simulink library "apCopterDragonfly_lib"  (R2018b)
settings: Solver=VariableStepAuto  StartTime=0.0  StopTime=10.0  RelTol=1e-3
undefined symbols (not defined in the file or in its folder): ap_dragonfly, DiscIntNeverNeededParam
libraries: simulink x2, cntrlAttiRedIndi_lib x2, cntrlPosNdi_lib x2, indi_lib x1, traj_lib x1, control_allocation_lib x1, ndi_lib x1, filters_lib x1, fmCopterAltHoldIndi_lib x1, axes_transformation_lib x1
settings Model: Creator=Ybeyer  LastModifiedBy=yannic
settings SFSimCC: SimUseLocalCustomCode=off
settings RTWCC: RTWUseLocalCustomCode=off
settings CodeAppCC: StateflowObjectComments=on

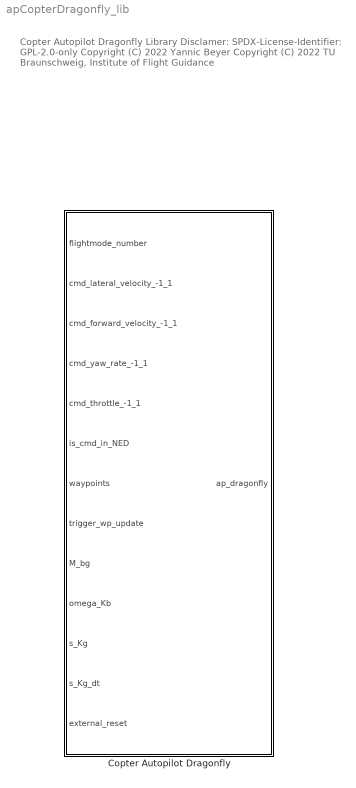
== system apCopterDragonfly_lib ==
  note: Copter Autopilot Dragonfly Library
      |
      | Disclamer:
      | SPDX-License-Identifier: GPL-2.0-only
      |
      | Copyright (C) 2022 Yannic Beyer
      | Copyright (C) 2022 TU Braunschweig, Institute of Flight Guidance
  Copter Autopilot Dragonfly : Subsystem  mask{fm=ap_dragonfly}
      mask prompts: fm "Dragonfly parameters struct, see apCopterDragonflyLoadParams"
      mask DialogControl DescGroupVar Prompt: Copter Autopilot Dragonfly
      mask DialogControl Control1 Prompt: flightmode numbers:
      mask DialogControl Control2 Prompt: loiter: 0
      mask DialogControl Control3 Prompt: guided: 1

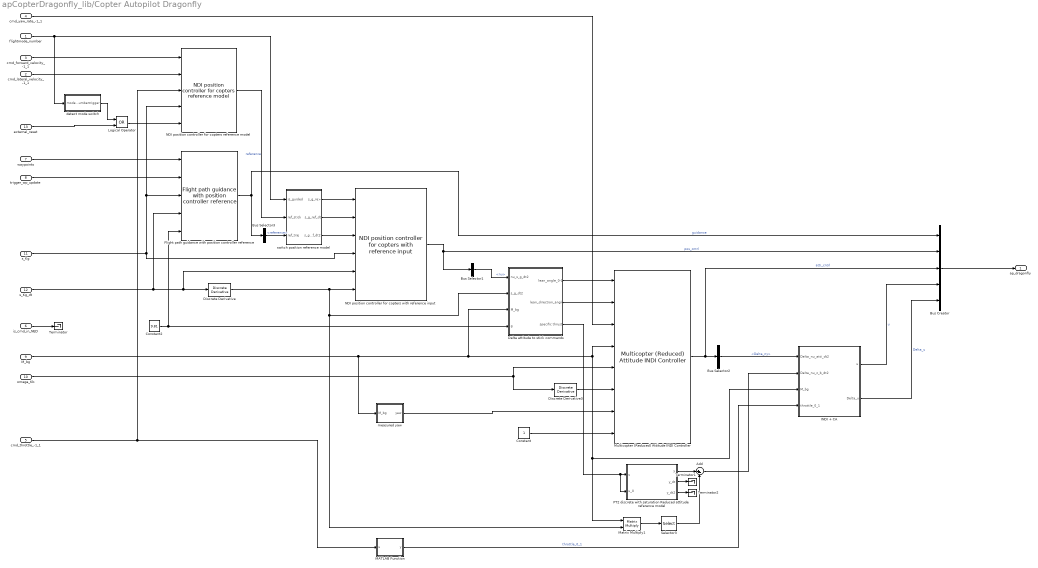
== system apCopterDragonfly_lib/Copter Autopilot Dragonfly ==
  flightmode_number : Inport  SampleTime=fm.sample_time
  cmd_lateral_velocity_-1_1 : Inport  Port=2  SampleTime=fm.sample_time
  cmd_forward_velocity_-1_1 : Inport  Port=3  SampleTime=fm.sample_time
  cmd_yaw_rate_-1_1 : Inport  Port=4  SampleTime=fm.sample_time
  cmd_throttle_-1_1 : Inport  Port=5  SampleTime=fm.sample_time
  is_cmd_in_NED : Inport  Port=6  SampleTime=fm.sample_time
  waypoints : Inport  Port=7
  trigger_wp_update : Inport  Port=8
  M_bg : Inport  Port=9  SampleTime=fm.sample_time
  omega_Kb : Inport  Port=10  SampleTime=fm.sample_time
  s_Kg : Inport  Port=11  SampleTime=fm.sample_time
  s_Kg_dt : Inport  Port=12  SampleTime=fm.sample_time
  external_reset : Inport  Port=13  SampleTime=fm.sample_time
  Add : Sum  Inputs=|+-
  Bus Creator : BusCreator  Inputs=5
  Bus Selector1 : BusSelector  OutputSignals=pseudo_control.nu
  Bus Selector2 : BusSelector  OutputSignals=pseudo_control.Delta_ny
  Bus Selector3 : BusSelector  OutputSignals=reference
  Constant : Constant
  Constant2 : Constant  Value=9.81
  Delta attitude to stick commands : Subsystem
  Discrete Derivative : simulink/Discrete/Discrete Derivative  gainval=1.0  ICPrevScaledInput=0.0  OutMin=[]  OutMax=[]  OutDataType=fixdt(1, 16)  OutScaling=2^-10  DoSatur=off
  Discrete Derivative3 : simulink/Discrete/Discrete Derivative  gainval=1.0  ICPrevScaledInput=0.0  OutMin=[]  OutMax=[]  OutDataType=fixdt(1, 16)  OutScaling=2^-10  DoSatur=off
  Flight path guidance with position controller reference : traj_lib/Flight path guidance with position controller reference  traj_params=fm.traj  T_inner_loop=2./fm.atc.rm.leanfreq + fm.motor_time_constant + 2./fm.sens_filt.omega
      settings: SourceProductName=LADAC
  INDI + CA : Subsystem
  Logical Operator : Logic  Operator=OR  AllPortsSameDT=off  OutDataTypeStr=boolean
  MATLAB Function : MATLAB Function  TreatAsAtomicUnit=on
  Matrix Multiply1 : Product  Multiplication=Matrix(*)
  Multicopter (Reduced) Attitude INDI Controller : cntrlAttiRedIndi_lib/Multicopter (Reduced) Attitude INDI Controller  atc=fm.atc  T=fm.motor_time_constant + 2./fm.sens_filt.omega
  NDI position controller for copters reference model : cntrlPosNdi_lib/NDI position controller for copters reference model  psc=fm.psc
      settings: SourceProductName=LADAC
  NDI position controller for copters with reference input : cntrlPosNdi_lib/NDI position controller for copters with reference input  psc=fm.psc  T_inner_loop=2./fm.atc.rm.leanfreq + fm.motor_time_constant + 2./fm.sens_filt.omega
      settings: SourceProductName=LADAC
  PT2 discrete with saturation Reduced attitude reference model : Subsystem  mask{omega=fm.atc.rm.leanfreq, d=fm.atc.rm.leandamp, x_dt2_max=inf, x_dt2_min=-inf, x_dt_max=inf, x_dt_min=-inf, x_max=inf, x_min=-inf, x_init=0, x_dt_init=0}
      mask prompts: omega "Natural frequency"; d "Damping ratio"; x_dt2_max "Maximum acceleration"; x_dt2_min "Minimum acceleration"; x_dt_max "Maximum rate"; x_dt_min "Minimum rate"; x_max "Maximum position"; x_min "Minimum position"; x_init "Initial position"; x_dt_init "Initial rate"
  Selector3 : Selector  InputPortWidth=3  IndexOptions=Index vector (dialog)  Indices=3  OutputSizes=1
  Terminator : Terminator
  Terminator1 : Terminator
  Terminator2 : Terminator
  detect mode switch : Subsystem
  measured yaw : Subsystem
  switch position reference model : Subsystem
  ap_dragonfly : Outport  SampleTime=fm.sample_time
  wires:
  waypoints/1 -> Flight path guidance with position controller reference/1
  cmd_lateral_velocity_-1_1/1 -> NDI position controller for copters reference model/2
  cmd_forward_velocity_-1_1/1 -> NDI position controller for copters reference model/1
  PT2 discrete with saturation Reduced attitude reference model/1(y) -> Add/1
  PT2 discrete with saturation Reduced attitude reference model/3(y_dt2) -> Terminator2/1
  PT2 discrete with saturation Reduced attitude reference model/2(y_dt) -> Terminator1/1
  Add/1 -> INDI + CA/2(Delta_nu_z_b_dt2)
  Bus Selector2/1 -> INDI + CA/1(Delta_nu_atti_dt2)  "<Delta_ny>"
  cmd_throttle_-1_1/1 -> NDI position controller for copters reference model/3, MATLAB Function/1(u)
  INDI + CA/2(Delta_u) -> Bus Creator/5  "Delta_u"
  INDI + CA/1(u) -> Bus Creator/4  "u"
  MATLAB Function/1(y) -> INDI + CA/4(throttle_0_1)  "throttle_0_1"
  Delta attitude to stick commands/1(lean_angle_0-1) -> Multicopter (Reduced) Attitude INDI Controller/1
  Delta attitude to stick commands/2(lean_direction_angle) -> Multicopter (Reduced) Attitude INDI Controller/2
  Discrete Derivative3/1 -> Multicopter (Reduced) Attitude INDI Controller/6
  Multicopter (Reduced) Attitude INDI Controller/1 -> Bus Creator/3, Bus Selector2/1  "atti_cntrl"
  is_cmd_in_NED/1 -> Terminator/1
  Bus Creator/1 -> ap_dragonfly/1
  Bus Selector1/1 -> Delta attitude to stick commands/1(nu_s_g_dt2)  "<nu>"
  measured yaw/1(yaw) -> Multicopter (Reduced) Attitude INDI Controller/7
  M_bg/1 -> measured yaw/1(M_bg), Delta attitude to stick commands/3(M_bg), INDI + CA/3(M_bg), Matrix Multiply1/1, Multicopter (Reduced) Attitude INDI Controller/4
  NDI position controller for copters with reference input/1 -> Bus Selector1/1, Bus Creator/2  "pos_cntrl"
  omega_Kb/1 -> Multicopter (Reduced) Attitude INDI Controller/5, Discrete Derivative3/1
  s_Kg/1 -> NDI position controller for copters reference model/4, Flight path guidance with position controller reference/3, NDI position controller for copters with reference input/4
  Constant/1 -> Multicopter (Reduced) Attitude INDI Controller/8
  cmd_yaw_rate_-1_1/1 -> Multicopter (Reduced) Attitude INDI Controller/3
  s_Kg_dt/1 -> Flight path guidance with position controller reference/4, Discrete Derivative/1, NDI position controller for copters with reference input/5
  Flight path guidance with position controller reference/1 -> Bus Creator/1, Bus Selector3/1  "guidance"
  switch position reference model/3(s_g_ref_dt2) -> NDI position controller for copters with reference input/3
  switch position reference model/2(s_g_ref_dt) -> NDI position controller for copters with reference input/2
  switch position reference model/1(s_g_re>) -> NDI position controller for copters with reference input/1
  Matrix Multiply1/1 -> Selector3/1
  Selector3/1 -> Add/2
  Delta attitude to stick commands/3(specific thrust) -> PT2 discrete with saturation Reduced attitude reference model/2(u_0), PT2 discrete with saturation Reduced attitude reference model/1(u)
  trigger_wp_update/1 -> Flight path guidance with position controller reference/2
  Discrete Derivative/1 -> Matrix Multiply1/2, Delta attitude to stick commands/2(s_g_dt2), NDI position controller for copters with reference input/6
  Constant2/1 -> Flight path guidance with position controller reference/5, Delta attitude to stick commands/4(g)
  NDI position controller for copters reference model/1 -> switch position reference model/2(ref_stick)  "reference"
  Bus Selector3/1 -> switch position reference model/3(ref_traj)  "<reference>"
  flightmode_number/1 -> detect mode switch/1(mode number), switch position reference model/1(is_guided)
  Logical Operator/1 -> NDI position controller for copters reference model/5
  detect mode switch/1(trigger) -> Logical Operator/1
  external_reset/1 -> Logical Operator/2

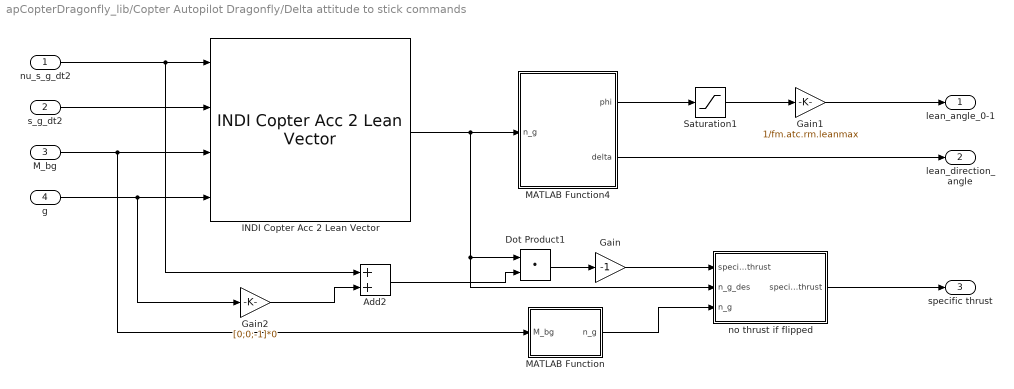
== system apCopterDragonfly_lib/Copter Autopilot Dragonfly/Delta attitude to stick commands ==
  nu_s_g_dt2 : Inport
  s_g_dt2 : Inport  Port=2
  M_bg : Inport  Port=3
  g : Inport  Port=4
  Add2 : Sum
  Dot Product1 : DotProduct  InputSameDT=on  OutDataTypeStr=Inherit: Inherit via internal rule
  Gain : Gain  Gain=-1
  Gain1 : Gain  Gain=1/fm.atc.rm.leanmax
  Gain2 : Gain  Gain=[0;0;-1]*0
  INDI Copter Acc 2 Lean Vector : indi_lib/INDI Copter Acc 2 Lean Vector  SystemSampleTime=-1
      settings: SourceProductName=LADAC
  MATLAB Function : MATLAB Function  TreatAsAtomicUnit=on
  MATLAB Function4 : MATLAB Function  TreatAsAtomicUnit=on
  Saturation1 : Saturate  UpperLimit=fm.atc.rm.leanmax  LowerLimit=0
  no thrust if flipped : MATLAB Function  TreatAsAtomicUnit=on
  lean_angle_0-1 : Outport
  lean_direction_angle : Outport  Port=2
  specific thrust : Outport  Port=3
  wires:
  MATLAB Function4/2(delta) -> lean_direction_angle/1
  Gain1/1 -> lean_angle_0-1/1
  nu_s_g_dt2/1 -> Add2/1, INDI Copter Acc 2 Lean Vector/1
  Saturation1/1 -> Gain1/1
  MATLAB Function4/1(phi) -> Saturation1/1
  g/1 -> Gain2/1, INDI Copter Acc 2 Lean Vector/4
  s_g_dt2/1 -> INDI Copter Acc 2 Lean Vector/2
  M_bg/1 -> MATLAB Function/1(M_bg), INDI Copter Acc 2 Lean Vector/3
  Dot Product1/1 -> Gain/1
  Gain/1 -> no thrust if flipped/1("specific_thrust ")
  INDI Copter Acc 2 Lean Vector/1 -> no thrust if flipped/2(n_g_des), Dot Product1/1, MATLAB Function4/1(n_g)
  Gain2/1 -> Add2/2
  Add2/1 -> Dot Product1/2
  no thrust if flipped/1(specific_thrust) -> specific thrust/1
  MATLAB Function/1(n_g) -> no thrust if flipped/3(n_g)

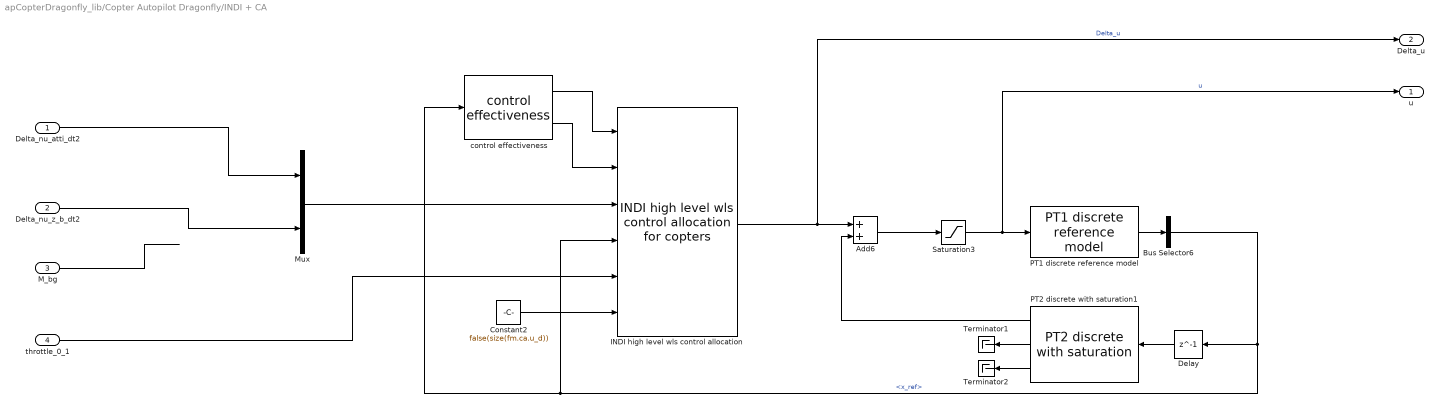
== system apCopterDragonfly_lib/Copter Autopilot Dragonfly/INDI + CA ==
  Delta_nu_atti_dt2 : Inport
  Delta_nu_z_b_dt2 : Inport  Port=2
  M_bg : Inport  Port=3
  throttle_0_1 : Inport  Port=4
  Add6 : Sum
  Bus Selector6 : BusSelector  OutputSignals=x_ref
  Constant2 : Constant  Value=false(size(fm.ca.u_d))
  Delay : Delay  DelayLength=1
  INDI high level wls control allocation : control_allocation_lib/INDI high level wls control allocation for copters  ca=fm.ca  is_Delta_W_v_check=off  is_W_check=off  is_iter_check=off
  Mux : Mux  Inputs=2
  PT1 discrete reference model : ndi_lib/PT1 discrete reference model  T=fm.motor_time_constant  x_max=inf  x_min=-inf  x_dt_max=inf  x_dt_min=-inf  x_init=0
      settings: SourceProductName=LADAC
  PT2 discrete with saturation1 : filters_lib/PT2 discrete with saturation  omega=fm.sens_filt.omega  d=fm.sens_filt.D  x_dt2_max=inf  x_dt2_min=-inf  x_dt_max=inf  x_dt_min=-inf  x_max=inf  x_min=-inf  x_init=0  x_dt_init=0
      settings: SourceProductName=LADAC
  Saturation3 : Saturate  UpperLimit=fm.ca.u_max  LowerLimit=fm.ca.u_min
  Terminator1 : Terminator
  Terminator2 : Terminator
  control effectiveness : fmCopterAltHoldIndi_lib/Multicopter Altitude Hold Flight Mode with INDI and reduced attitude control/control effectiveness  SystemSampleTime=-1
      settings: SourceProductName=LADAC
  u : Outport
  Delta_u : Outport  Port=2  PortDimensions=4
  wires:
  control effectiveness/2 -> INDI high level wls control allocation/2
  M_bg/1 -> ?
  Delta_nu_z_b_dt2/1 -> Mux/2
  Delta_nu_atti_dt2/1 -> Mux/1
  Add6/1 -> Saturation3/1
  PT1 discrete reference model/1 -> Bus Selector6/1
  PT2 discrete with saturation1/3 -> Terminator2/1
  PT2 discrete with saturation1/2 -> Terminator1/1
  Constant2/1 -> INDI high level wls control allocation/6
  control effectiveness/1 -> INDI high level wls control allocation/1
  Bus Selector6/1 -> INDI high level wls control allocation/4, control effectiveness/1, Delay/1  "<x_ref>"
  throttle_0_1/1 -> INDI high level wls control allocation/5
  Delay/1 -> PT2 discrete with saturation1/1
  INDI high level wls control allocation/1 -> Add6/1, Delta_u/1  "Delta_u"
  Saturation3/1 -> PT1 discrete reference model/1, u/1  "u"
  Mux/1 -> INDI high level wls control allocation/3
  PT2 discrete with saturation1/1 -> Add6/2

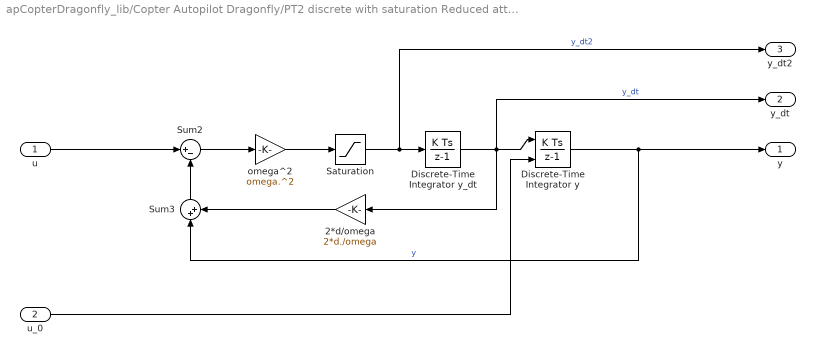
== system apCopterDragonfly_lib/Copter Autopilot Dragonfly/PT2 discrete with saturation Reduced attitude reference model ==
  u : Inport
  u_0 : Inport  Port=2
  2*d/omega : Gain  Gain=2*d./omega
  Discrete-Time Integrator y : DiscreteIntegrator  InitialConditionSource=external  InitialCondition=x_init  SampleTime=-1  OutDataTypeStr=Inherit: Inherit via back propagation  LimitOutput=on  UpperSaturationLimit=x_max  LowerSaturationLimit=x_min  ICPrevOutput=DiscIntNeverNeededParam  ICPrevScaledInput=DiscIntNeverNeededParam
  Discrete-Time Integrator y_dt : DiscreteIntegrator  InitialCondition=x_dt_init  SampleTime=-1  OutDataTypeStr=Inherit: Inherit via back propagation  LimitOutput=on  UpperSaturationLimit=x_dt_max  LowerSaturationLimit=x_dt_min  ICPrevOutput=DiscIntNeverNeededParam  ICPrevScaledInput=DiscIntNeverNeededParam
  Saturation : Saturate  UpperLimit=x_dt2_max  LowerLimit=x_dt2_min
  Sum2 : Sum  Inputs=|+-
  Sum3 : Sum  Inputs=|++
  omega^2 : Gain  Gain=omega.^2
  y : Outport
  y_dt : Outport  Port=2
  y_dt2 : Outport  Port=3
  wires:
  Saturation/1 -> y_dt2/1, Discrete-Time Integrator y_dt/1  "y_dt2"
  omega^2/1 -> Saturation/1
  Sum3/1 -> Sum2/2
  u/1 -> Sum2/1
  2*d/omega/1 -> Sum3/2
  Sum2/1 -> omega^2/1
  Discrete-Time Integrator y/1 -> Sum3/1, y/1  "y"
  Discrete-Time Integrator y_dt/1 -> 2*d/omega/1, y_dt/1, Discrete-Time Integrator y/1  "y_dt"
  u_0/1 -> Discrete-Time Integrator y/2

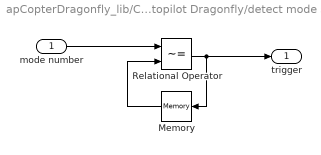
== system apCopterDragonfly_lib/Copter Autopilot Dragonfly/detect mode switch ==
  mode number : Inport
  Memory : Memory
  Relational Operator : RelationalOperator  Operator=~=  OutDataTypeStr=boolean  RndMeth=Simplest
  trigger : Outport
  wires:
  Relational Operator/1 -> Memory/1, trigger/1
  Memory/1 -> Relational Operator/2
  mode number/1 -> Relational Operator/1

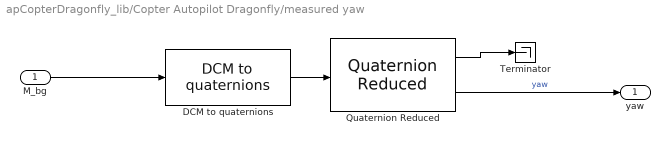
== system apCopterDragonfly_lib/Copter Autopilot Dragonfly/measured yaw ==
  M_bg : Inport
  DCM to quaternions : axes_transformation_lib/DCM to quaternions  SystemSampleTime=-1
      settings: SourceProductName=LADAC
  Quaternion Reduced : cntrlAttiRedIndi_lib/Multicopter (Reduced) Attitude INDI Controller/measure/Quaternion Reduced  SystemSampleTime=-1
  Terminator : Terminator
  yaw : Outport
  wires:
  DCM to quaternions/1 -> Quaternion Reduced/1
  Quaternion Reduced/1 -> Terminator/1
  Quaternion Reduced/2 -> yaw/1  "yaw"
  M_bg/1 -> DCM to quaternions/1

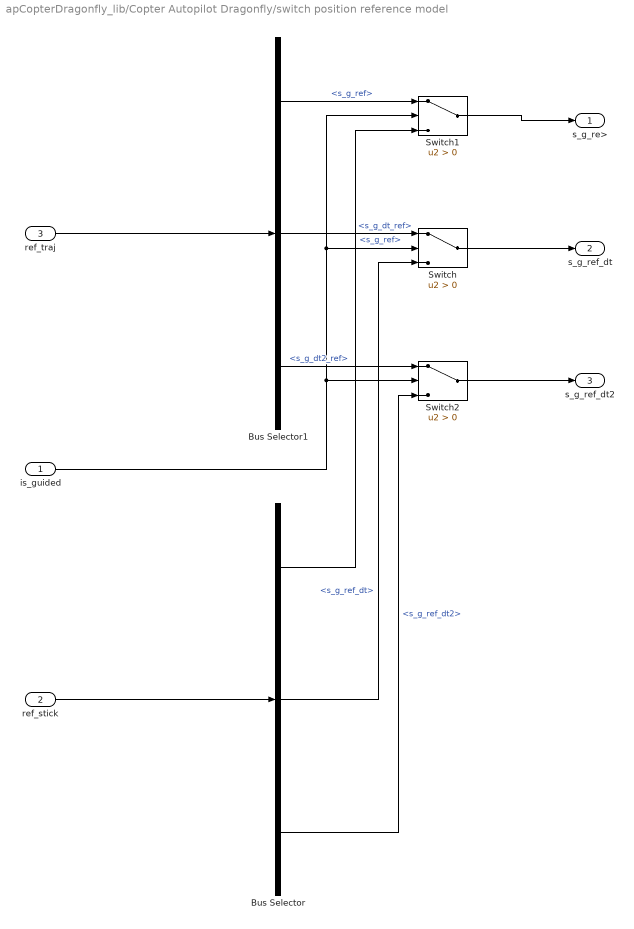
== system apCopterDragonfly_lib/Copter Autopilot Dragonfly/switch position reference model ==
  is_guided : Inport
  ref_stick : Inport  Port=2
  ref_traj : Inport  Port=3
  Bus Selector : BusSelector  OutputSignals=s_g_ref,s_g_ref_dt,s_g_ref_dt2
  Bus Selector1 : BusSelector  OutputSignals=s_g_ref,s_g_dt_ref,s_g_dt2_ref
  Switch : Switch  Criteria=u2 > Threshold
  Switch1 : Switch  Criteria=u2 > Threshold
  Switch2 : Switch  Criteria=u2 > Threshold
  s_g_re> : Outport
  s_g_ref_dt : Outport  Port=2
  s_g_ref_dt2 : Outport  Port=3
  wires:
  Bus Selector/1 -> Switch1/3  "<s_g_ref>"
  ref_stick/1 -> Bus Selector/1
  Bus Selector/2 -> Switch/3  "<s_g_ref_dt>"
  Bus Selector/3 -> Switch2/3  "<s_g_ref_dt2>"
  ref_traj/1 -> Bus Selector1/1
  Switch/1 -> s_g_ref_dt/1
  Bus Selector1/2 -> Switch/1  "<s_g_dt_ref>"
  is_guided/1 -> Switch2/2, Switch1/2, Switch/2
  Bus Selector1/1 -> Switch1/1  "<s_g_ref>"
  Bus Selector1/3 -> Switch2/1  "<s_g_dt2_ref>"
  Switch1/1 -> s_g_re>/1
  Switch2/1 -> s_g_ref_dt2/1

== matlab function apCopterDragonfly_lib/Copter Autopilot Dragonfly/Delta attitude to stick commands/MATLAB Function ==
  data: M_bg input; n_g output
function n_g = fcn(M_bg)
n_g = dcm2LeanVector(M_bg);
end

== matlab function apCopterDragonfly_lib/Copter Autopilot Dragonfly/Delta attitude to stick commands/MATLAB Function4 ==
  data: n_g input; phi output; delta output
function [phi,delta] = leanVector2LeanAngles(n_g)
[phi,delta] = leanVector2LeanAngles(n_g);
end

== matlab function apCopterDragonfly_lib/Copter Autopilot Dragonfly/Delta attitude to stick commands/no thrust if flipped ==
  data: specific_thrust input; n_g_des input; specific_thrust output; n_g input
function specific_thrust = fcn(specific_thrust,n_g_des,n_g)
proj = dot(n_g,n_g_des);
if proj < 0
    specific_thrust(:) = -specific_thrust;
end
end

== matlab function apCopterDragonfly_lib/Copter Autopilot Dragonfly/MATLAB Function ==
  data: u input; y output
function y = fcn(u)
y = 0.5*u+0.5;
